simulink model "cacc_consensus_test_u0"  (R2022b)
settings: Solver=VariableStepAuto  StartTime=0.0  StopTime=60  RelTol=1e-3
undefined symbols (not defined in the file): A, B, C, D, K_cacc
libraries: cstblocks x4, simulink x1
settings Model: Creator=phatdo  LastModifiedBy=phatdo
settings DataIOCC: ReturnWorkspaceOutputs=off

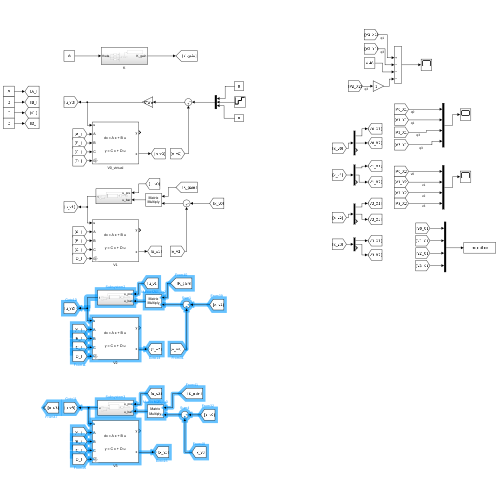
[thumbnail: Simulink's stored preview of the top-level diagram]
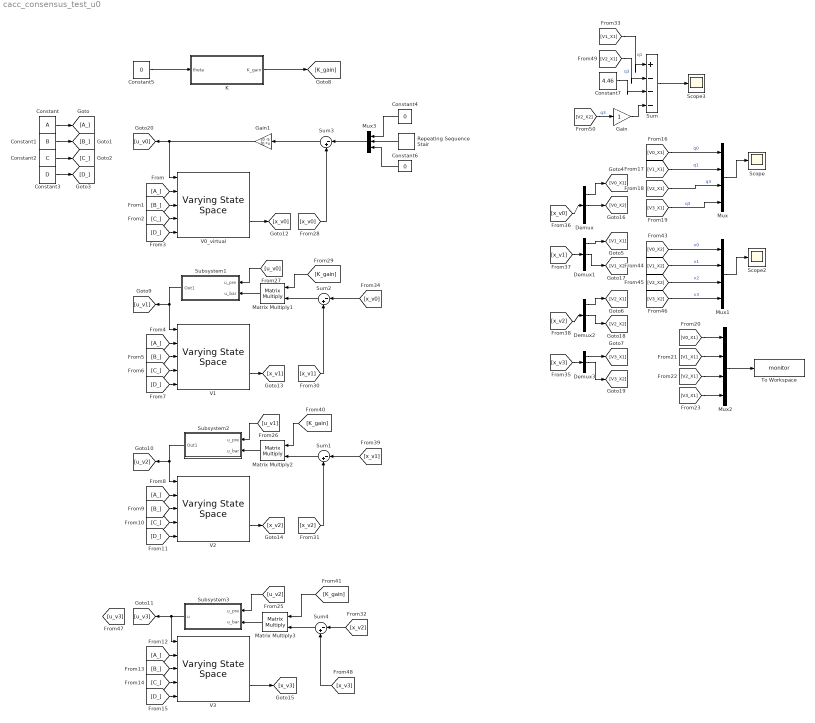
== system cacc_consensus_test_u0 ==
  Constant : Constant  Value=A
  Constant1 : Constant  Value=B
  Constant2 : Constant  Value=C
  Constant3 : Constant  Value=D
  Constant4 : Constant  Value=0
  Constant5 : Constant  Value=0
  Constant6 : Constant  Value=0
  Constant7 : Constant  Value=4.46
  Demux{,1..3} (4 alike) : Demux  Outputs=3
  Gain : Gain
  Gain1 : Gain  Gain=[0 -5 0]  Multiplication=Matrix(K*u) (u vector)
  K : Subsystem
  Matrix Multiply1 : Product  Multiplication=Matrix(*)
  Matrix Multiply2 : Product  Multiplication=Matrix(*)
  Matrix Multiply3 : Product  Multiplication=Matrix(*)
  Mux : Mux
  Mux1 : Mux
  Mux2 : Mux
  Mux3 : Mux  Inputs=3
  Repeating Sequence Stair : simulink/Sources/Repeating Sequence Stair  OutValues=[20 40 60]  tsamp=20  OutMin=[]  OutMax=[]  OutDataTypeStr=double  OutputDataTypeScalingMode=double  OutDataType=fixdt(0,8)  ConRadixGroup=Best Precision: Vector-wise  OutScaling=2^-12
  Scope : Scope
  Scope2 : Scope
  Scope3 : Scope
  Subsystem1 : Subsystem
  Subsystem2 : Subsystem
  Subsystem3 : Subsystem
  Sum : Sum  Inputs=|+---
  Sum{1..4} (4 alike) : Sum  Inputs=|-+
  To Workspace : ToWorkspace  VariableName=monitor  SaveFormat=Timeseries  SampleTime=-1
  V0_virtual : cstblocks/Linear Parameter Varying/Varying State Space  x0=[0;0;0]  xNames=''  OutputX=on  OutputDX=off
  V1 : cstblocks/Linear Parameter Varying/Varying State Space  x0=[0;0;0]  xNames=''  OutputX=on  OutputDX=off
  V2 : cstblocks/Linear Parameter Varying/Varying State Space  x0=[0;0;0]  xNames=''  OutputX=on  OutputDX=off
  V3 : cstblocks/Linear Parameter Varying/Varying State Space  x0=[0 ;0 ; 0]  xNames=''  OutputX=on  OutputDX=off
  wires:
  Sum2/1 -> Matrix Multiply1/2
  Sum1/1 -> Matrix Multiply2/2
  Constant2/1 -> [C_]
  Constant/1 -> [A_]
  Constant3/1 -> [D_]
  Constant1/1 -> [B_]
  [B_] -> V0_virtual/3
  [A_] -> V0_virtual/2
  [C_] -> V0_virtual/4
  [D_] -> V0_virtual/5
  [D_] -> V1/5
  [A_] -> V2/2
  [A_] -> V3/2
  [A_] -> V1/2
  [B_] -> V1/3
  [C_] -> V1/4
  [B_] -> V2/3
  [C_] -> V2/4
  [D_] -> V2/5
  [B_] -> V3/3
  [C_] -> V3/4
  [D_] -> V3/5
  [V2_X1] -> Mux/3  "q3"
  [V3_X1] -> Mux/4  "q3"
  Mux/1 -> Scope/1
  [V1_X1] -> Mux/2  "q1"
  [V0_X1] -> Mux/1  "q0"
  Constant5/1 -> K/1(theta)
  [V1_X1] -> Mux2/2
  [V0_X1] -> Mux2/1
  [V3_X1] -> Mux2/4
  Mux2/1 -> To Workspace/1
  [V2_X1] -> Mux2/3
  K/1(K_gain) -> [K_gain]
  Gain1/1 -> [u_v0], V0_virtual/1
  Subsystem1/1(Out1) -> V1/1, [u_v1]
  Subsystem2/1(Out1) -> [u_v2], V2/1
  Subsystem3/1(u) -> V3/1, [u_v3]
  [u_v0] -> Subsystem1/1(u_pre)
  [u_v1] -> Subsystem2/1(u_pre)
  [u_v2] -> Subsystem3/1(u_pre)
  V0_virtual/2 -> [x_v0]
  Matrix Multiply1/1 -> Subsystem1/2(u_bar)
  [K_gain] -> Matrix Multiply1/1
  V1/2 -> [x_v1]
  [x_v1] -> Sum2/2
  Matrix Multiply2/1 -> Subsystem2/2(u_bar)
  V2/2 -> [x_v2]
  [x_v2] -> Sum1/2
  V3/2 -> [x_v3]
  [x_v0] -> Sum2/1
  [x_v1] -> Sum1/1
  [x_v0] -> Demux/1
  [x_v1] -> Demux1/1
  [x_v2] -> Demux2/1
  [x_v3] -> Demux3/1
  [K_gain] -> Matrix Multiply2/1
  Matrix Multiply3/1 -> Subsystem3/2(u_bar)
  [K_gain] -> Matrix Multiply3/1
  Demux/1 -> [V0_X1]
  Demux1/1 -> [V1_X1]
  Demux2/1 -> [V2_X1]
  Demux3/1 -> [V3_X1]
  Demux/2 -> [V0_X2]
  [V0_X2] -> Mux1/1  "v0"
  Mux1/1 -> Scope2/1
  [V3_X2] -> Mux1/4  "v3"
  Demux1/2 -> [V1_X2]
  [V1_X2] -> Mux1/2  "v1"
  Demux2/2 -> [V2_X2]
  Demux3/2 -> [V3_X2]
  [V2_X2] -> Mux1/3  "v2"
  [x_v3] -> Sum4/2
  Sum4/1 -> Matrix Multiply3/2
  [x_v2] -> Sum4/1
  [V1_X1] -> Sum/1  "q1"
  [V2_X1] -> Sum/2  "q3"
  Constant7/1 -> Sum/3
  Gain/1 -> Sum/4
  Sum/1 -> Scope3/1
  [V2_X2] -> Gain/1  "q3"
  [x_v0] -> Sum3/2
  Sum3/1 -> Gain1/1
  Mux3/1 -> Sum3/1
  Repeating Sequence Stair/1 -> Mux3/2
  Constant4/1 -> Mux3/1
  Constant6/1 -> Mux3/3

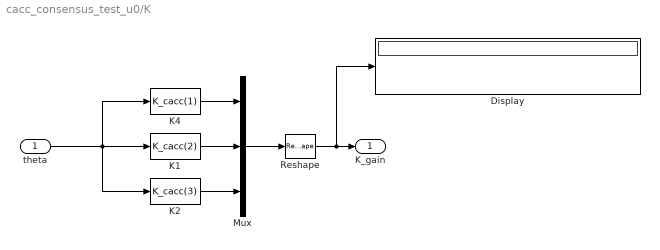
== system cacc_consensus_test_u0/K ==
  theta : Inport
  Display : Display
  K1 : Fcn  Expr=K_cacc(2)
  K2 : Fcn  Expr=K_cacc(3)
  K4 : Fcn  Expr=K_cacc(1)
  Mux : Mux  Inputs=3
  Reshape : Reshape  OutputDimensionality=Customize  OutputDimensions=[1,3]
  K_gain : Outport
  wires:
  Mux/1 -> Reshape/1
  Reshape/1 -> Display/1, K_gain/1
  K4/1 -> Mux/1
  K1/1 -> Mux/2
  K2/1 -> Mux/3
  theta/1 -> K2/1, K1/1, K4/1

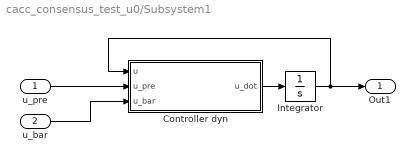
== system cacc_consensus_test_u0/Subsystem1 ==
  u_pre : Inport
  u_bar : Inport  Port=2
  Controller dyn : MATLAB Function  TreatAsAtomicUnit=on
  Integrator : Integrator
  Out1 : Outport
  wires:
  Controller dyn/1(u_dot) -> Integrator/1
  Integrator/1 -> Controller dyn/1(u), Out1/1
  u_pre/1 -> Controller dyn/2(u_pre)
  u_bar/1 -> Controller dyn/3(u_bar)

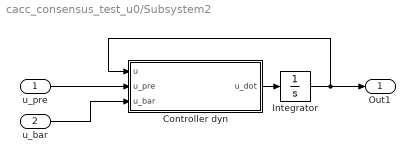
== system cacc_consensus_test_u0/Subsystem2 ==
  u_pre : Inport
  u_bar : Inport  Port=2
  Controller dyn : MATLAB Function  TreatAsAtomicUnit=on
  Integrator : Integrator
  Out1 : Outport
  wires:
  Controller dyn/1(u_dot) -> Integrator/1
  Integrator/1 -> Controller dyn/1(u), Out1/1
  u_pre/1 -> Controller dyn/2(u_pre)
  u_bar/1 -> Controller dyn/3(u_bar)

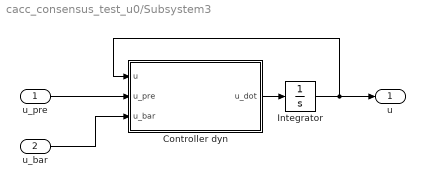
== system cacc_consensus_test_u0/Subsystem3 ==
  u_pre : Inport
  u_bar : Inport  Port=2
  Controller dyn : MATLAB Function  TreatAsAtomicUnit=on
  Integrator : Integrator
  u : Outport
  wires:
  Controller dyn/1(u_dot) -> Integrator/1
  Integrator/1 -> Controller dyn/1(u), u/1
  u_pre/1 -> Controller dyn/2(u_pre)
  u_bar/1 -> Controller dyn/3(u_bar)

== matlab function cacc_consensus_test_u0/Subsystem1/Controller dyn ==
  data: u input; u_dot output; u_pre input; u_bar input
function u_dot = cacc(u, u_pre, u_bar)

h = 1; % second

u_dot = -1/h * u + 1/h * (u_pre - u_bar);

end

== matlab function cacc_consensus_test_u0/Subsystem2/Controller dyn ==
  data: u input; u_dot output; u_pre input; u_bar input
function u_dot = cacc(u, u_pre, u_bar)

h = 1; % second

u_dot = -1/h * u + 1/h * (u_pre - u_bar);

end

== matlab function cacc_consensus_test_u0/Subsystem3/Controller dyn ==
  data: u input; u_dot output; u_pre input; u_bar input
function u_dot = cacc(u, u_pre, u_bar)

h = 1; % second

u_dot = -1/h * u + 1/h * (u_pre - u_bar);

end
